simulink model "B"  (R2024a)
settings: Solver=VariableStepAuto  StartTime=0.0  StopTime=10*10^-6  RelTol=1e-3
undefined symbols (not defined in the file): c1, c3, rxDpIndex
libraries: commblkcod2 x64, commofdm x64, commdigbbndam3 x64, commsink2 x1, commseqgen3 x1
(part 1 of 3)
settings Model: Creator=Honest  LastModifiedBy=NEYMAR
settings RTWCC: GPUComputeCapability=3.5

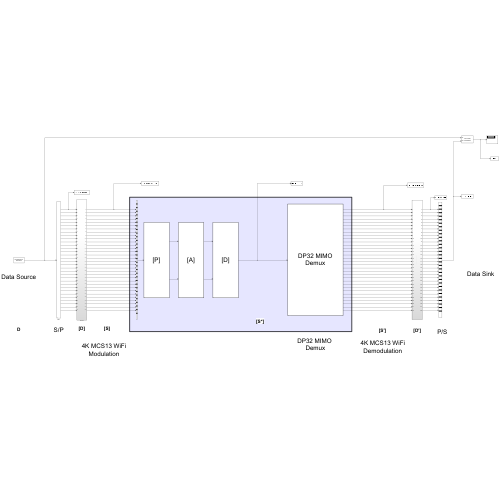
[thumbnail: Simulink's stored preview of the top-level diagram]
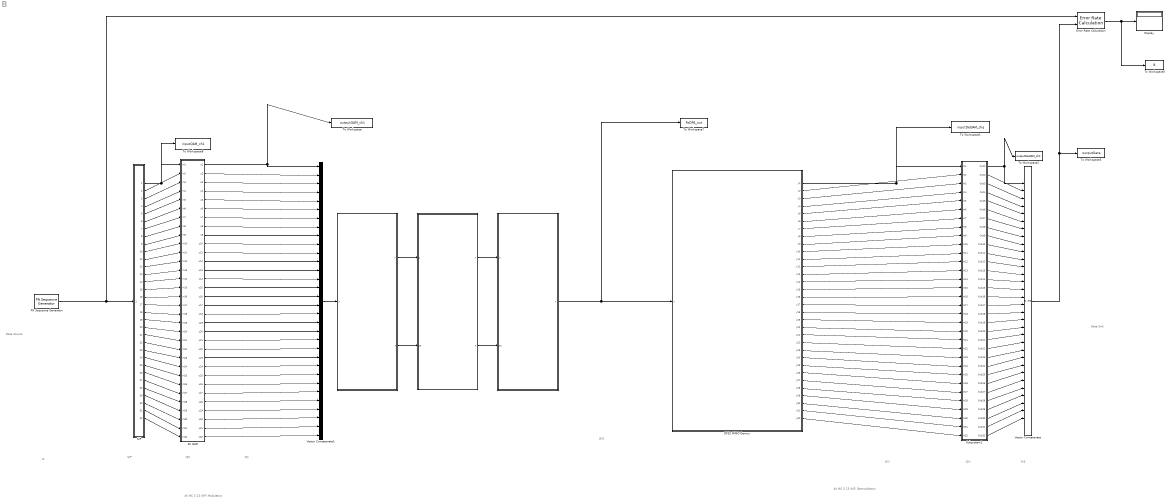
== system B ==
  note: Data Source
  note: D
  note: Data Sink
  note: S/P
  note: 4K MC S 13 WiFi Modulation
  note: P/S
  note: [S']
  note: [D]
  note: [S]
  note: [S*]
  note: [D']
  note: 4K MC S 13 WiFi Demodulation
  " " : MATLAB Function  TreatAsAtomicUnit=on
  " " : MATLAB Function  TreatAsAtomicUnit=on
  " DP32 MIMO Demux" : MATLAB Function  TreatAsAtomicUnit=on
  "    " : MATLAB Function  TreatAsAtomicUnit=on
  4K QAM : Subsystem
  Display : Display
  Error Rate Calculation : commsink2/Error Rate Calculation  N=0  st_delay=0  cp_mode=Entire frame  subframe=[]  PMode=Port  WsName=ErrorVec  RsMode2=off  stop=off  numErr=10000  maxBits=1e8
  PN Sequence Generator : commseqgen3/PN Sequence Generator  poly='z^15 + z^14 + 1'  ini_sta=[0 0 0 0 0 0 0 0 0 0 0 0 0 0 1]  outBitMaskSource=Dialog parameter  shift=0  outVarSiz=off  maxOutSizeMode=Dialog parameter  maxOutSize=[10 1]  Ts=1.0845987*10^-11  sampPerFrame=1254400  reset=off  bitPackedOutputs=off  outDataType=double  numPackedBits=8  bitPackDataSigned=off  bitPackedOutDType=double
  S/P : Subsystem
      mask Display: text(5, 10, 'Serial to Parallel Converter');
  Subsystem1 : Subsystem
  To Workspace : ToWorkspace  VariableName=outputQAM_ch1  SampleTime=-1
      settings: Save2DSignal=2-D array (concatenate along first dimension)
  To Workspace1 : ToWorkspace  VariableName=inputDeQAM_chq  SampleTime=-1
      settings: Save2DSignal=2-D array (concatenate along first dimension)
  To Workspace2 : ToWorkspace  VariableName=outputDeQAM_ch1  SampleTime=-1
      settings: Save2DSignal=2-D array (concatenate along first dimension)
  To Workspace3 : ToWorkspace  VariableName=outputData  SampleTime=-1
      settings: Save2DSignal=2-D array (concatenate along first dimension)
  To Workspace5 : ToWorkspace  VariableName=B  SampleTime=-1
      settings: MaxDataPoints=1  Save2DSignal=2-D array (concatenate along first dimension)
  To Workspace7 : ToWorkspace  VariableName=RxDPA_out  SampleTime=-1
      settings: Save2DSignal=2-D array (concatenate along first dimension)
  To Workspace8 : ToWorkspace  VariableName=inputQAM_ch1  SampleTime=-1
      settings: Save2DSignal=2-D array (concatenate along first dimension)
  Vector Concatenate : Concatenate  NumInputs=32
  Vector Concatenate1 : Concatenate  NumInputs=32
  wires:
  S/P/9(Out9) -> 4K QAM/9(In9)
  4K QAM/23(u23) -> Vector Concatenate1/23
  S/P/17(Out17) -> 4K QAM/17(In17)
  Subsystem1/18(Out18) -> Vector Concatenate/18
  S/P/18(Out18) -> 4K QAM/18(In18)
  Vector Concatenate1/1 -> " "/1(u)
  Subsystem1/12(Out12) -> Vector Concatenate/12
  4K QAM/20(u20) -> Vector Concatenate1/20
  S/P/32(Out32) -> 4K QAM/32(In32)
  Subsystem1/7(Out7) -> Vector Concatenate/7
  Subsystem1/1(Out1) -> Vector Concatenate/1, To Workspace2/1
  Subsystem1/30(Out30) -> Vector Concatenate/30
  4K QAM/26(u26) -> Vector Concatenate1/26
  4K QAM/18(u18) -> Vector Concatenate1/18
  Subsystem1/23(Out23) -> Vector Concatenate/23
  S/P/12(Out12) -> 4K QAM/12(In12)
  4K QAM/19(u19) -> Vector Concatenate1/19
  Subsystem1/26(Out26) -> Vector Concatenate/26
  4K QAM/32(u32) -> Vector Concatenate1/32
  4K QAM/30(u30) -> Vector Concatenate1/30
  4K QAM/28(u28) -> Vector Concatenate1/28
  S/P/13(Out13) -> 4K QAM/13(In13)
  Subsystem1/25(Out25) -> Vector Concatenate/25
  Subsystem1/10(Out10) -> Vector Concatenate/10
  Subsystem1/24(Out24) -> Vector Concatenate/24
  S/P/8(Out8) -> 4K QAM/8(In8)
  Subsystem1/29(Out29) -> Vector Concatenate/29
  Subsystem1/21(Out21) -> Vector Concatenate/21
  Subsystem1/27(Out27) -> Vector Concatenate/27
  Subsystem1/22(Out22) -> Vector Concatenate/22
  4K QAM/31(u31) -> Vector Concatenate1/31
  Subsystem1/28(Out28) -> Vector Concatenate/28
  Subsystem1/32(Out32) -> Vector Concatenate/32
  Subsystem1/6(Out6) -> Vector Concatenate/6
  Subsystem1/20(Out20) -> Vector Concatenate/20
  Subsystem1/8(Out8) -> Vector Concatenate/8
  S/P/21(Out21) -> 4K QAM/21(In21)
  Subsystem1/19(Out19) -> Vector Concatenate/19
  S/P/2(Out2) -> 4K QAM/2(In2)
  Subsystem1/3(Out3) -> Vector Concatenate/3
  Subsystem1/11(Out11) -> Vector Concatenate/11
  Subsystem1/4(Out4) -> Vector Concatenate/4
  S/P/20(Out20) -> 4K QAM/20(In20)
  Subsystem1/13(Out13) -> Vector Concatenate/13
  S/P/29(Out29) -> 4K QAM/29(In29)
  4K QAM/29(u29) -> Vector Concatenate1/29
  S/P/14(Out14) -> 4K QAM/14(In14)
  Subsystem1/14(Out14) -> Vector Concatenate/14
  Subsystem1/9(Out9) -> Vector Concatenate/9
  S/P/23(Out23) -> 4K QAM/23(In23)
  S/P/19(Out19) -> 4K QAM/19(In19)
  Subsystem1/31(Out31) -> Vector Concatenate/31
  S/P/26(Out26) -> 4K QAM/26(In26)
  4K QAM/17(u17) -> Vector Concatenate1/17
  S/P/25(Out25) -> 4K QAM/25(In25)
  S/P/6(Out6) -> 4K QAM/6(In6)
  S/P/22(Out22) -> 4K QAM/22(In22)
  Subsystem1/16(Out16) -> Vector Concatenate/16
  S/P/28(Out28) -> 4K QAM/28(In28)
  S/P/31(Out31) -> 4K QAM/31(In31)
  S/P/27(Out27) -> 4K QAM/27(In27)
  S/P/16(Out16) -> 4K QAM/16(In16)
  Subsystem1/5(Out5) -> Vector Concatenate/5
  S/P/15(Out15) -> 4K QAM/15(In15)
  S/P/10(Out10) -> 4K QAM/10(In10)
  Subsystem1/15(Out15) -> Vector Concatenate/15
  S/P/24(Out24) -> 4K QAM/24(In24)
  S/P/30(Out30) -> 4K QAM/30(In30)
  S/P/3(Out3) -> 4K QAM/3(In3)
  S/P/7(Out7) -> 4K QAM/7(In7)
  S/P/1(Out1) -> 4K QAM/1(In1), To Workspace8/1
  4K QAM/21(u21) -> Vector Concatenate1/21
  S/P/4(Out4) -> 4K QAM/4(In4)
  S/P/5(Out5) -> 4K QAM/5(In5)
  Subsystem1/17(Out17) -> Vector Concatenate/17
  S/P/11(Out11) -> 4K QAM/11(In11)
  Subsystem1/2(Out2) -> Vector Concatenate/2
  Vector Concatenate/1 -> Error Rate Calculation/2, To Workspace3/1
  Error Rate Calculation/1 -> Display/1, To Workspace5/1
  PN Sequence Generator/1 -> Error Rate Calculation/1, S/P/1(In1)
  " DP32 MIMO Demux"/2(y2) -> Subsystem1/2(In2)
  " DP32 MIMO Demux"/3(y3) -> Subsystem1/3(In3)
  " DP32 MIMO Demux"/4(y4) -> Subsystem1/4(In4)
  " DP32 MIMO Demux"/5(y5) -> Subsystem1/5(In5)
  " DP32 MIMO Demux"/6(y6) -> Subsystem1/6(In6)
  " DP32 MIMO Demux"/7(y7) -> Subsystem1/7(In7)
  " DP32 MIMO Demux"/8(y8) -> Subsystem1/8(In8)
  " DP32 MIMO Demux"/9(y9) -> Subsystem1/9(In9)
  " DP32 MIMO Demux"/10(y10) -> Subsystem1/10(In10)
  " DP32 MIMO Demux"/11(y11) -> Subsystem1/11(In11)
  " DP32 MIMO Demux"/12(y12) -> Subsystem1/12(In12)
  " DP32 MIMO Demux"/13(y13) -> Subsystem1/13(In13)
  " DP32 MIMO Demux"/14(y14) -> Subsystem1/14(In14)
  " DP32 MIMO Demux"/15(y15) -> Subsystem1/15(In15)
  " DP32 MIMO Demux"/16(y16) -> Subsystem1/16(In16)
  " DP32 MIMO Demux"/17(y17) -> Subsystem1/17(In17)
  " DP32 MIMO Demux"/18(y18) -> Subsystem1/18(In18)
  " DP32 MIMO Demux"/19(y19) -> Subsystem1/19(In19)
  " DP32 MIMO Demux"/20(y20) -> Subsystem1/20(In20)
  " DP32 MIMO Demux"/21(y21) -> Subsystem1/21(In21)
  " DP32 MIMO Demux"/22(y22) -> Subsystem1/22(In22)
  " DP32 MIMO Demux"/23(y23) -> Subsystem1/23(In23)
  " DP32 MIMO Demux"/24(y24) -> Subsystem1/24(In24)
  " DP32 MIMO Demux"/25(y25) -> Subsystem1/25(In25)
  " DP32 MIMO Demux"/26(y26) -> Subsystem1/26(In26)
  " DP32 MIMO Demux"/27(y27) -> Subsystem1/27(In27)
  " DP32 MIMO Demux"/28(y28) -> Subsystem1/28(In28)
  " DP32 MIMO Demux"/29(y29) -> Subsystem1/29(In29)
  " DP32 MIMO Demux"/30(y30) -> Subsystem1/30(In30)
  " DP32 MIMO Demux"/31(y31) -> Subsystem1/31(In31)
  " DP32 MIMO Demux"/32(y32) -> Subsystem1/32(In32)
  4K QAM/2(u2) -> Vector Concatenate1/2
  4K QAM/5(u5) -> Vector Concatenate1/5
  4K QAM/6(u6) -> Vector Concatenate1/6
  4K QAM/7(u7) -> Vector Concatenate1/7
  4K QAM/8(u8) -> Vector Concatenate1/8
  4K QAM/9(u9) -> Vector Concatenate1/9
  4K QAM/10(u10) -> Vector Concatenate1/10
  4K QAM/11(u11) -> Vector Concatenate1/11
  4K QAM/12(u12) -> Vector Concatenate1/12
  4K QAM/13(u13) -> Vector Concatenate1/13
  4K QAM/14(u14) -> Vector Concatenate1/14
  4K QAM/15(u15) -> Vector Concatenate1/15
  4K QAM/16(u16) -> Vector Concatenate1/16
  4K QAM/24(u24) -> Vector Concatenate1/24
  4K QAM/3(u3) -> Vector Concatenate1/3
  4K QAM/4(u4) -> Vector Concatenate1/4
  4K QAM/22(u22) -> Vector Concatenate1/22
  4K QAM/25(u25) -> Vector Concatenate1/25
  4K QAM/27(u27) -> Vector Concatenate1/27
  " DP32 MIMO Demux"/1(y1) -> Subsystem1/1(In1), To Workspace1/1
  4K QAM/1(u1) -> To Workspace/1, Vector Concatenate1/1
  " "/1(y) -> "    "/1(u)
  "    "/1(y) -> " "/1(u)
  " "/1(y) -> To Workspace7/1, " DP32 MIMO Demux"/1(u)
  " "/2(s) -> "    "/2(ss)
  "    "/2(s) -> " "/2(ss)

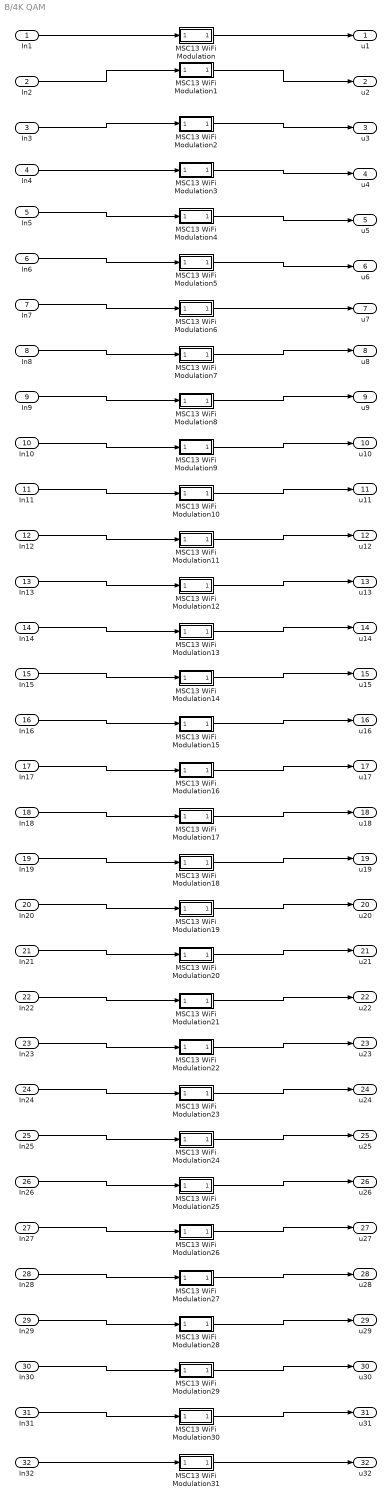
== system B/4K QAM ==
  In1 : Inport
  In2 : Inport  Port=2
  In3 : Inport  Port=3
  In4 : Inport  Port=4
  In5 : Inport  Port=5
  In6 : Inport  Port=6
  In7 : Inport  Port=7
  In8 : Inport  Port=8
  In9 : Inport  Port=9
  In10 : Inport  Port=10
  In11 : Inport  Port=11
  In12 : Inport  Port=12
  In13 : Inport  Port=13
  In14 : Inport  Port=14
  In15 : Inport  Port=15
  In16 : Inport  Port=16
  In17 : Inport  Port=17
  In18 : Inport  Port=18
  In19 : Inport  Port=19
  In20 : Inport  Port=20
  In21 : Inport  Port=21
  In22 : Inport  Port=22
  In23 : Inport  Port=23
  In24 : Inport  Port=24
  In25 : Inport  Port=25
  In26 : Inport  Port=26
  In27 : Inport  Port=27
  In28 : Inport  Port=28
  In29 : Inport  Port=29
  In30 : Inport  Port=30
  In31 : Inport  Port=31
  In32 : Inport  Port=32
  MSC13 WiFi Modulation : Subsystem
  MSC13 WiFi Modulation1 : Subsystem
  MSC13 WiFi Modulation10 : Subsystem
  MSC13 WiFi Modulation11 : Subsystem
  MSC13 WiFi Modulation12 : Subsystem
  MSC13 WiFi Modulation13 : Subsystem
  MSC13 WiFi Modulation14 : Subsystem
  MSC13 WiFi Modulation15 : Subsystem
  MSC13 WiFi Modulation16 : Subsystem
  MSC13 WiFi Modulation17 : Subsystem
  MSC13 WiFi Modulation18 : Subsystem
  MSC13 WiFi Modulation19 : Subsystem
  MSC13 WiFi Modulation2 : Subsystem
  MSC13 WiFi Modulation20 : Subsystem
  MSC13 WiFi Modulation21 : Subsystem
  MSC13 WiFi Modulation22 : Subsystem
  MSC13 WiFi Modulation23 : Subsystem
  MSC13 WiFi Modulation24 : Subsystem
  MSC13 WiFi Modulation25 : Subsystem
  MSC13 WiFi Modulation26 : Subsystem
  MSC13 WiFi Modulation27 : Subsystem
  MSC13 WiFi Modulation28 : Subsystem
  MSC13 WiFi Modulation29 : Subsystem
  MSC13 WiFi Modulation3 : Subsystem
  MSC13 WiFi Modulation30 : Subsystem
  MSC13 WiFi Modulation31 : Subsystem
  MSC13 WiFi Modulation4 : Subsystem
  MSC13 WiFi Modulation5 : Subsystem
  MSC13 WiFi Modulation6 : Subsystem
  MSC13 WiFi Modulation7 : Subsystem
  MSC13 WiFi Modulation8 : Subsystem
  MSC13 WiFi Modulation9 : Subsystem
  u1 : Outport
  u2 : Outport  Port=2
  u3 : Outport  Port=3
  u4 : Outport  Port=4
  u5 : Outport  Port=5
  u6 : Outport  Port=6
  u7 : Outport  Port=7
  u8 : Outport  Port=8
  u9 : Outport  Port=9
  u10 : Outport  Port=10
  u11 : Outport  Port=11
  u12 : Outport  Port=12
  u13 : Outport  Port=13
  u14 : Outport  Port=14
  u15 : Outport  Port=15
  u16 : Outport  Port=16
  u17 : Outport  Port=17
  u18 : Outport  Port=18
  u19 : Outport  Port=19
  u20 : Outport  Port=20
  u21 : Outport  Port=21
  u22 : Outport  Port=22
  u23 : Outport  Port=23
  u24 : Outport  Port=24
  u25 : Outport  Port=25
  u26 : Outport  Port=26
  u27 : Outport  Port=27
  u28 : Outport  Port=28
  u29 : Outport  Port=29
  u30 : Outport  Port=30
  u31 : Outport  Port=31
  u32 : Outport  Port=32
  wires:
  In1/1 -> MSC13 WiFi Modulation/1(In1)
  MSC13 WiFi Modulation/1(Out1) -> u1/1
  In2/1 -> MSC13 WiFi Modulation1/1(In1)
  MSC13 WiFi Modulation1/1(Out1) -> u2/1
  In32/1 -> MSC13 WiFi Modulation31/1(In1)
  In31/1 -> MSC13 WiFi Modulation30/1(In1)
  In30/1 -> MSC13 WiFi Modulation29/1(In1)
  In27/1 -> MSC13 WiFi Modulation26/1(In1)
  In28/1 -> MSC13 WiFi Modulation27/1(In1)
  In29/1 -> MSC13 WiFi Modulation28/1(In1)
  In26/1 -> MSC13 WiFi Modulation25/1(In1)
  In25/1 -> MSC13 WiFi Modulation24/1(In1)
  In24/1 -> MSC13 WiFi Modulation23/1(In1)
  In23/1 -> MSC13 WiFi Modulation22/1(In1)
  In22/1 -> MSC13 WiFi Modulation21/1(In1)
  In21/1 -> MSC13 WiFi Modulation20/1(In1)
  In20/1 -> MSC13 WiFi Modulation19/1(In1)
  In19/1 -> MSC13 WiFi Modulation18/1(In1)
  In18/1 -> MSC13 WiFi Modulation17/1(In1)
  In17/1 -> MSC13 WiFi Modulation16/1(In1)
  In16/1 -> MSC13 WiFi Modulation15/1(In1)
  In15/1 -> MSC13 WiFi Modulation14/1(In1)
  In14/1 -> MSC13 WiFi Modulation13/1(In1)
  In13/1 -> MSC13 WiFi Modulation12/1(In1)
  In12/1 -> MSC13 WiFi Modulation11/1(In1)
  In11/1 -> MSC13 WiFi Modulation10/1(In1)
  In10/1 -> MSC13 WiFi Modulation9/1(In1)
  In9/1 -> MSC13 WiFi Modulation8/1(In1)
  In8/1 -> MSC13 WiFi Modulation7/1(In1)
  In7/1 -> MSC13 WiFi Modulation6/1(In1)
  In6/1 -> MSC13 WiFi Modulation5/1(In1)
  In4/1 -> MSC13 WiFi Modulation3/1(In1)
  In3/1 -> MSC13 WiFi Modulation2/1(In1)
  In5/1 -> MSC13 WiFi Modulation4/1(In1)
  MSC13 WiFi Modulation2/1(Out1) -> u3/1
  MSC13 WiFi Modulation3/1(Out1) -> u4/1
  MSC13 WiFi Modulation5/1(Out1) -> u6/1
  MSC13 WiFi Modulation4/1(Out1) -> u5/1
  MSC13 WiFi Modulation6/1(Out1) -> u7/1
  MSC13 WiFi Modulation7/1(Out1) -> u8/1
  MSC13 WiFi Modulation8/1(Out1) -> u9/1
  MSC13 WiFi Modulation9/1(Out1) -> u10/1
  MSC13 WiFi Modulation10/1(Out1) -> u11/1
  MSC13 WiFi Modulation11/1(Out1) -> u12/1
  MSC13 WiFi Modulation12/1(Out1) -> u13/1
  MSC13 WiFi Modulation13/1(Out1) -> u14/1
  MSC13 WiFi Modulation14/1(Out1) -> u15/1
  MSC13 WiFi Modulation15/1(Out1) -> u16/1
  MSC13 WiFi Modulation16/1(Out1) -> u17/1
  MSC13 WiFi Modulation17/1(Out1) -> u18/1
  MSC13 WiFi Modulation18/1(Out1) -> u19/1
  MSC13 WiFi Modulation19/1(Out1) -> u20/1
  MSC13 WiFi Modulation20/1(Out1) -> u21/1
  MSC13 WiFi Modulation21/1(Out1) -> u22/1
  MSC13 WiFi Modulation22/1(Out1) -> u23/1
  MSC13 WiFi Modulation23/1(Out1) -> u24/1
  MSC13 WiFi Modulation24/1(Out1) -> u25/1
  MSC13 WiFi Modulation25/1(Out1) -> u26/1
  MSC13 WiFi Modulation26/1(Out1) -> u27/1
  MSC13 WiFi Modulation27/1(Out1) -> u28/1
  MSC13 WiFi Modulation28/1(Out1) -> u29/1
  MSC13 WiFi Modulation29/1(Out1) -> u30/1
  MSC13 WiFi Modulation30/1(Out1) -> u31/1
  MSC13 WiFi Modulation31/1(Out1) -> u32/1

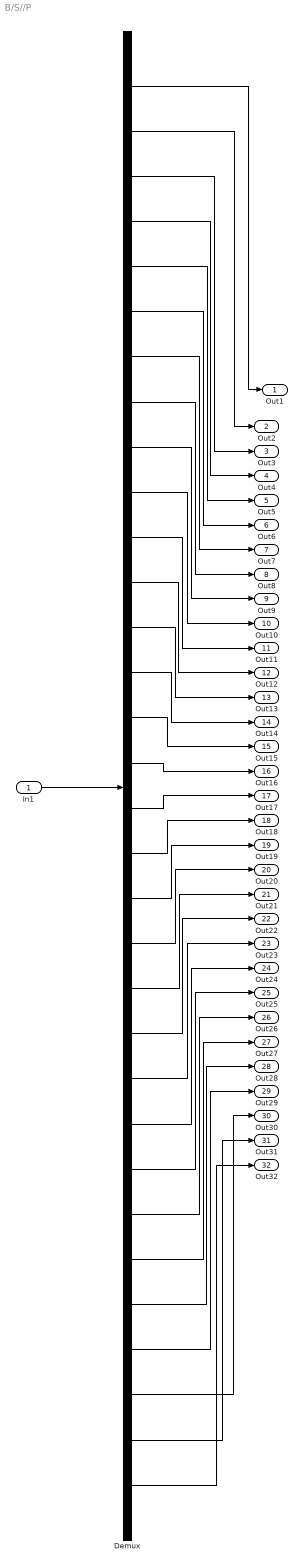
== system B/S//P ==
  In1 : Inport
  Demux : Demux  Outputs=32
  Out1 : Outport
  Out2 : Outport  Port=2
  Out3 : Outport  Port=3
  Out4 : Outport  Port=4
  Out5 : Outport  Port=5
  Out6 : Outport  Port=6
  Out7 : Outport  Port=7
  Out8 : Outport  Port=8
  Out9 : Outport  Port=9
  Out10 : Outport  Port=10
  Out11 : Outport  Port=11
  Out12 : Outport  Port=12
  Out13 : Outport  Port=13
  Out14 : Outport  Port=14
  Out15 : Outport  Port=15
  Out16 : Outport  Port=16
  Out17 : Outport  Port=17
  Out18 : Outport  Port=18
  Out19 : Outport  Port=19
  Out20 : Outport  Port=20
  Out21 : Outport  Port=21
  Out22 : Outport  Port=22
  Out23 : Outport  Port=23
  Out24 : Outport  Port=24
  Out25 : Outport  Port=25
  Out26 : Outport  Port=26
  Out27 : Outport  Port=27
  Out28 : Outport  Port=28
  Out29 : Outport  Port=29
  Out30 : Outport  Port=30
  Out31 : Outport  Port=31
  Out32 : Outport  Port=32
  wires:
  Demux/28 -> Out28/1
  Demux/2 -> Out2/1
  Demux/16 -> Out16/1
  In1/1 -> Demux/1
  Demux/13 -> Out13/1
  Demux/6 -> Out6/1
  Demux/7 -> Out7/1
  Demux/21 -> Out21/1
  Demux/3 -> Out3/1
  Demux/11 -> Out11/1
  Demux/1 -> Out1/1
  Demux/20 -> Out20/1
  Demux/5 -> Out5/1
  Demux/4 -> Out4/1
  Demux/8 -> Out8/1
  Demux/9 -> Out9/1
  Demux/12 -> Out12/1
  Demux/14 -> Out14/1
  Demux/29 -> Out29/1
  Demux/15 -> Out15/1
  Demux/17 -> Out17/1
  Demux/18 -> Out18/1
  Demux/10 -> Out10/1
  Demux/22 -> Out22/1
  Demux/19 -> Out19/1
  Demux/23 -> Out23/1
  Demux/30 -> Out30/1
  Demux/27 -> Out27/1
  Demux/25 -> Out25/1
  Demux/26 -> Out26/1
  Demux/24 -> Out24/1
  Demux/31 -> Out31/1
  Demux/32 -> Out32/1

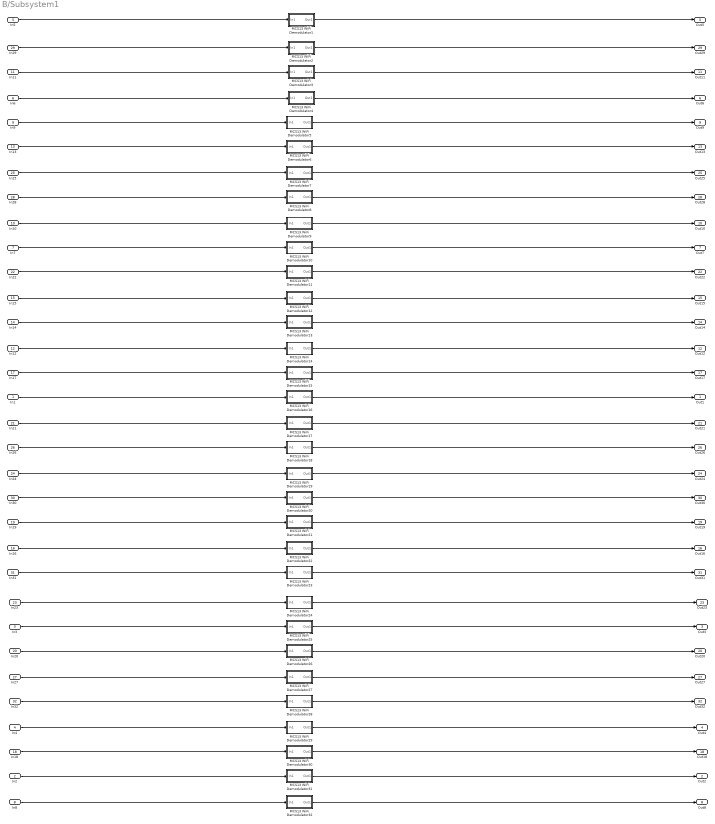
== system B/Subsystem1 ==
  In1 : Inport
  In2 : Inport  Port=2
  In3 : Inport  Port=3
  In4 : Inport  Port=4
  In5 : Inport  Port=5
  In6 : Inport  Port=6
  In7 : Inport  Port=7
  In8 : Inport  Port=8
  In9 : Inport  Port=9
  In10 : Inport  Port=10
  In11 : Inport  Port=11
  In12 : Inport  Port=12
  In13 : Inport  Port=13
  In14 : Inport  Port=14
  In15 : Inport  Port=15
  In16 : Inport  Port=16
  In17 : Inport  Port=17
  In18 : Inport  Port=18
  In19 : Inport  Port=19
  In20 : Inport  Port=20
  In21 : Inport  Port=21
  In22 : Inport  Port=22
  In23 : Inport  Port=23
  In24 : Inport  Port=24
  In25 : Inport  Port=25
  In26 : Inport  Port=26
  In27 : Inport  Port=27
  In28 : Inport  Port=28
  In29 : Inport  Port=29
  In30 : Inport  Port=30
  In31 : Inport  Port=31
  In32 : Inport  Port=32
  MCS13 WiFi Demodulator1 : Subsystem
  MCS13 WiFi Demodulator10 : Subsystem
  MCS13 WiFi Demodulator11 : Subsystem
  MCS13 WiFi Demodulator12 : Subsystem
  MCS13 WiFi Demodulator13 : Subsystem
  MCS13 WiFi Demodulator14 : Subsystem
  MCS13 WiFi Demodulator15 : Subsystem
  MCS13 WiFi Demodulator16 : Subsystem
  MCS13 WiFi Demodulator17 : Subsystem
  MCS13 WiFi Demodulator18 : Subsystem
  MCS13 WiFi Demodulator19 : Subsystem
  MCS13 WiFi Demodulator2 : Subsystem
  MCS13 WiFi Demodulator20 : Subsystem
  MCS13 WiFi Demodulator21 : Subsystem
  MCS13 WiFi Demodulator22 : Subsystem
  MCS13 WiFi Demodulator23 : Subsystem
  MCS13 WiFi Demodulator24 : Subsystem
  MCS13 WiFi Demodulator25 : Subsystem
  MCS13 WiFi Demodulator26 : Subsystem
  MCS13 WiFi Demodulator27 : Subsystem
  MCS13 WiFi Demodulator28 : Subsystem
  MCS13 WiFi Demodulator29 : Subsystem
  MCS13 WiFi Demodulator3 : Subsystem
  MCS13 WiFi Demodulator30 : Subsystem
  MCS13 WiFi Demodulator31 : Subsystem
  MCS13 WiFi Demodulator32 : Subsystem
  MCS13 WiFi Demodulator4 : Subsystem
  MCS13 WiFi Demodulator5 : Subsystem
  MCS13 WiFi Demodulator6 : Subsystem
  MCS13 WiFi Demodulator7 : Subsystem
  MCS13 WiFi Demodulator8 : Subsystem
  MCS13 WiFi Demodulator9 : Subsystem
  Out1 : Outport
  Out2 : Outport  Port=2
  Out3 : Outport  Port=3
  Out4 : Outport  Port=4
  Out5 : Outport  Port=5
  Out6 : Outport  Port=6
  Out7 : Outport  Port=7
  Out8 : Outport  Port=8
  Out9 : Outport  Port=9
  Out10 : Outport  Port=10
  Out11 : Outport  Port=11
  Out12 : Outport  Port=12
  Out13 : Outport  Port=13
  Out14 : Outport  Port=14
  Out15 : Outport  Port=15
  Out16 : Outport  Port=16
  Out17 : Outport  Port=17
  Out18 : Outport  Port=18
  Out19 : Outport  Port=19
  Out20 : Outport  Port=20
  Out21 : Outport  Port=21
  Out22 : Outport  Port=22
  Out23 : Outport  Port=23
  Out24 : Outport  Port=24
  Out25 : Outport  Port=25
  Out26 : Outport  Port=26
  Out27 : Outport  Port=27
  Out28 : Outport  Port=28
  Out29 : Outport  Port=29
  Out30 : Outport  Port=30
  Out31 : Outport  Port=31
  Out32 : Outport  Port=32
  wires:
  MCS13 WiFi Demodulator16/1(Out1) -> Out1/1
  MCS13 WiFi Demodulator31/1(Out1) -> Out2/1
  MCS13 WiFi Demodulator25/1(Out1) -> Out3/1
  MCS13 WiFi Demodulator29/1(Out1) -> Out4/1
  MCS13 WiFi Demodulator1/1(Out1) -> Out5/1
  MCS13 WiFi Demodulator4/1(Out1) -> Out6/1
  MCS13 WiFi Demodulator10/1(Out1) -> Out7/1
  MCS13 WiFi Demodulator32/1(Out1) -> Out8/1
  MCS13 WiFi Demodulator5/1(Out1) -> Out9/1
  MCS13 WiFi Demodulator9/1(Out1) -> Out10/1
  MCS13 WiFi Demodulator3/1(Out1) -> Out11/1
  MCS13 WiFi Demodulator14/1(Out1) -> Out12/1
  MCS13 WiFi Demodulator6/1(Out1) -> Out13/1
  MCS13 WiFi Demodulator13/1(Out1) -> Out14/1
  MCS13 WiFi Demodulator12/1(Out1) -> Out15/1
  MCS13 WiFi Demodulator22/1(Out1) -> Out16/1
  MCS13 WiFi Demodulator15/1(Out1) -> Out17/1
  MCS13 WiFi Demodulator30/1(Out1) -> Out18/1
  MCS13 WiFi Demodulator21/1(Out1) -> Out19/1
  MCS13 WiFi Demodulator26/1(Out1) -> Out20/1
  MCS13 WiFi Demodulator17/1(Out1) -> Out21/1
  MCS13 WiFi Demodulator11/1(Out1) -> Out22/1
  MCS13 WiFi Demodulator24/1(Out1) -> Out23/1
  MCS13 WiFi Demodulator19/1(Out1) -> Out24/1
  MCS13 WiFi Demodulator7/1(Out1) -> Out25/1
  MCS13 WiFi Demodulator18/1(Out1) -> Out26/1
  MCS13 WiFi Demodulator27/1(Out1) -> Out27/1
  MCS13 WiFi Demodulator8/1(Out1) -> Out28/1
  MCS13 WiFi Demodulator2/1(Out1) -> Out29/1
  MCS13 WiFi Demodulator20/1(Out1) -> Out30/1
  MCS13 WiFi Demodulator23/1(Out1) -> Out31/1
  MCS13 WiFi Demodulator28/1(Out1) -> Out32/1
  In19/1 -> MCS13 WiFi Demodulator21/1(In1)
  In3/1 -> MCS13 WiFi Demodulator25/1(In1)
  In31/1 -> MCS13 WiFi Demodulator23/1(In1)
  In2/1 -> MCS13 WiFi Demodulator31/1(In1)
  In13/1 -> MCS13 WiFi Demodulator6/1(In1)
  In1/1 -> MCS13 WiFi Demodulator16/1(In1)
  In18/1 -> MCS13 WiFi Demodulator30/1(In1)
  In10/1 -> MCS13 WiFi Demodulator9/1(In1)
  In4/1 -> MCS13 WiFi Demodulator29/1(In1)
  In5/1 -> MCS13 WiFi Demodulator1/1(In1)
  In28/1 -> MCS13 WiFi Demodulator8/1(In1)
  In21/1 -> MCS13 WiFi Demodulator17/1(In1)
  In14/1 -> MCS13 WiFi Demodulator13/1(In1)
  In15/1 -> MCS13 WiFi Demodulator12/1(In1)
  In20/1 -> MCS13 WiFi Demodulator26/1(In1)
  In11/1 -> MCS13 WiFi Demodulator3/1(In1)
  In22/1 -> MCS13 WiFi Demodulator11/1(In1)
  In7/1 -> MCS13 WiFi Demodulator10/1(In1)
  In23/1 -> MCS13 WiFi Demodulator24/1(In1)
  In12/1 -> MCS13 WiFi Demodulator14/1(In1)
  In30/1 -> MCS13 WiFi Demodulator20/1(In1)
  In9/1 -> MCS13 WiFi Demodulator5/1(In1)
  In32/1 -> MCS13 WiFi Demodulator28/1(In1)
  In29/1 -> MCS13 WiFi Demodulator2/1(In1)
  In16/1 -> MCS13 WiFi Demodulator22/1(In1)
  In26/1 -> MCS13 WiFi Demodulator18/1(In1)
  In24/1 -> MCS13 WiFi Demodulator19/1(In1)
  In25/1 -> MCS13 WiFi Demodulator7/1(In1)
  In8/1 -> MCS13 WiFi Demodulator32/1(In1)
  In6/1 -> MCS13 WiFi Demodulator4/1(In1)
  In27/1 -> MCS13 WiFi Demodulator27/1(In1)
  In17/1 -> MCS13 WiFi Demodulator15/1(In1)

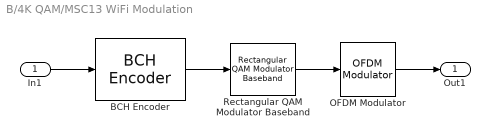
== system B/4K QAM/MSC13 WiFi Modulation ==
  In1 : Inport
  BCH Encoder : commblkcod2/BCH Encoder  n=47040  k=39200  specShortening=off  shortenedK=5  specGenPoly=off  genPoly='X^10 + X^8 + X^5 + X^4 + X^2 + X + 1'  specPrimPoly=off  prPoly='X^4 + X + 1'  specDisableGenCheck=off  specPuncture=off  punctVec=[ones(8,1); zeros(2,1)]
  OFDM Modulator : commofdm/OFDM Modulator  StatePerturbationForJacobian=1.0e-05  FFTLength=4096  NumGuardBandCarriers=[88; 88]  InsertDCNull=off  PilotInputPort=off  PilotCarrierIndices=[52;104;156;208;260]  CyclicPrefixLength=0  Windowing=off  WindowLength=1  OversamplingFactor=1  NumSymbols=1  NumTransmitAntennas=1  SimulateUsing=Interpreted execution
  Rectangular QAM Modulator Baseband : commdigbbndam3/Rectangular QAM Modulator Baseband  M=4096  InType=Bit  Enc=Gray  Mapping=[0:15]  PowType=Min. distance between symbols  MinDist=2  AvgPow=1  PeakPow=1  Ph=0  outDtype=double  outWordLen=16  outUDDataType=sfix(16)  outFracLenMode=Best precision  outFracLen=15  outDataTypeStr=double  outLastDataTypeStr=double
  Out1 : Outport
  wires:
  Rectangular QAM Modulator Baseband/1 -> OFDM Modulator/1
  OFDM Modulator/1 -> Out1/1
  BCH Encoder/1 -> Rectangular QAM Modulator Baseband/1
  In1/1 -> BCH Encoder/1

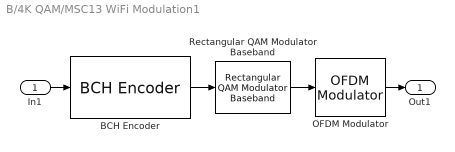
== system B/4K QAM/MSC13 WiFi Modulation1 ==
  In1 : Inport
  BCH Encoder : commblkcod2/BCH Encoder  n=47040  k=39200  specShortening=off  shortenedK=5  specGenPoly=off  genPoly='X^10 + X^8 + X^5 + X^4 + X^2 + X + 1'  specPrimPoly=off  prPoly='X^4 + X + 1'  specDisableGenCheck=off  specPuncture=off  punctVec=[ones(8,1); zeros(2,1)]
  OFDM Modulator : commofdm/OFDM Modulator  StatePerturbationForJacobian=1.0e-05  FFTLength=4096  NumGuardBandCarriers=[88; 88]  InsertDCNull=off  PilotInputPort=off  PilotCarrierIndices=[52;104;156;208;260]  CyclicPrefixLength=0  Windowing=off  WindowLength=1  OversamplingFactor=1  NumSymbols=1  NumTransmitAntennas=1  SimulateUsing=Interpreted execution
  Rectangular QAM Modulator Baseband : commdigbbndam3/Rectangular QAM Modulator Baseband  M=4096  InType=Bit  Enc=Gray  Mapping=[0:15]  PowType=Min. distance between symbols  MinDist=2  AvgPow=1  PeakPow=1  Ph=0  outDtype=double  outWordLen=16  outUDDataType=sfix(16)  outFracLenMode=Best precision  outFracLen=15  outDataTypeStr=double  outLastDataTypeStr=double
  Out1 : Outport
  wires:
  Rectangular QAM Modulator Baseband/1 -> OFDM Modulator/1
  OFDM Modulator/1 -> Out1/1
  BCH Encoder/1 -> Rectangular QAM Modulator Baseband/1
  In1/1 -> BCH Encoder/1

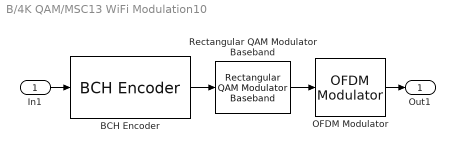
== system B/4K QAM/MSC13 WiFi Modulation10 ==
  In1 : Inport
  BCH Encoder : commblkcod2/BCH Encoder  n=47040  k=39200  specShortening=off  shortenedK=5  specGenPoly=off  genPoly='X^10 + X^8 + X^5 + X^4 + X^2 + X + 1'  specPrimPoly=off  prPoly='X^4 + X + 1'  specDisableGenCheck=off  specPuncture=off  punctVec=[ones(8,1); zeros(2,1)]
  OFDM Modulator : commofdm/OFDM Modulator  StatePerturbationForJacobian=1.0e-05  FFTLength=4096  NumGuardBandCarriers=[88; 88]  InsertDCNull=off  PilotInputPort=off  PilotCarrierIndices=[52;104;156;208;260]  CyclicPrefixLength=0  Windowing=off  WindowLength=1  OversamplingFactor=1  NumSymbols=1  NumTransmitAntennas=1  SimulateUsing=Interpreted execution
  Rectangular QAM Modulator Baseband : commdigbbndam3/Rectangular QAM Modulator Baseband  M=4096  InType=Bit  Enc=Gray  Mapping=[0:15]  PowType=Min. distance between symbols  MinDist=2  AvgPow=1  PeakPow=1  Ph=0  outDtype=double  outWordLen=16  outUDDataType=sfix(16)  outFracLenMode=Best precision  outFracLen=15  outDataTypeStr=double  outLastDataTypeStr=double
  Out1 : Outport
  wires:
  Rectangular QAM Modulator Baseband/1 -> OFDM Modulator/1
  OFDM Modulator/1 -> Out1/1
  BCH Encoder/1 -> Rectangular QAM Modulator Baseband/1
  In1/1 -> BCH Encoder/1

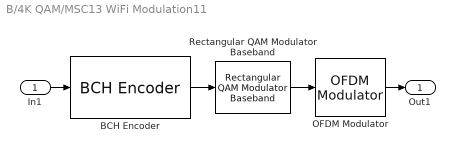
== system B/4K QAM/MSC13 WiFi Modulation11 ==
  In1 : Inport
  BCH Encoder : commblkcod2/BCH Encoder  n=47040  k=39200  specShortening=off  shortenedK=5  specGenPoly=off  genPoly='X^10 + X^8 + X^5 + X^4 + X^2 + X + 1'  specPrimPoly=off  prPoly='X^4 + X + 1'  specDisableGenCheck=off  specPuncture=off  punctVec=[ones(8,1); zeros(2,1)]
  OFDM Modulator : commofdm/OFDM Modulator  StatePerturbationForJacobian=1.0e-05  FFTLength=4096  NumGuardBandCarriers=[88; 88]  InsertDCNull=off  PilotInputPort=off  PilotCarrierIndices=[52;104;156;208;260]  CyclicPrefixLength=0  Windowing=off  WindowLength=1  OversamplingFactor=1  NumSymbols=1  NumTransmitAntennas=1  SimulateUsing=Interpreted execution
  Rectangular QAM Modulator Baseband : commdigbbndam3/Rectangular QAM Modulator Baseband  M=4096  InType=Bit  Enc=Gray  Mapping=[0:15]  PowType=Min. distance between symbols  MinDist=2  AvgPow=1  PeakPow=1  Ph=0  outDtype=double  outWordLen=16  outUDDataType=sfix(16)  outFracLenMode=Best precision  outFracLen=15  outDataTypeStr=double  outLastDataTypeStr=double
  Out1 : Outport
  wires:
  Rectangular QAM Modulator Baseband/1 -> OFDM Modulator/1
  OFDM Modulator/1 -> Out1/1
  BCH Encoder/1 -> Rectangular QAM Modulator Baseband/1
  In1/1 -> BCH Encoder/1

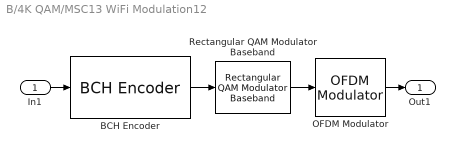
== system B/4K QAM/MSC13 WiFi Modulation12 ==
  In1 : Inport
  BCH Encoder : commblkcod2/BCH Encoder  n=47040  k=39200  specShortening=off  shortenedK=5  specGenPoly=off  genPoly='X^10 + X^8 + X^5 + X^4 + X^2 + X + 1'  specPrimPoly=off  prPoly='X^4 + X + 1'  specDisableGenCheck=off  specPuncture=off  punctVec=[ones(8,1); zeros(2,1)]
  OFDM Modulator : commofdm/OFDM Modulator  StatePerturbationForJacobian=1.0e-05  FFTLength=4096  NumGuardBandCarriers=[88; 88]  InsertDCNull=off  PilotInputPort=off  PilotCarrierIndices=[52;104;156;208;260]  CyclicPrefixLength=0  Windowing=off  WindowLength=1  OversamplingFactor=1  NumSymbols=1  NumTransmitAntennas=1  SimulateUsing=Interpreted execution
  Rectangular QAM Modulator Baseband : commdigbbndam3/Rectangular QAM Modulator Baseband  M=4096  InType=Bit  Enc=Gray  Mapping=[0:15]  PowType=Min. distance between symbols  MinDist=2  AvgPow=1  PeakPow=1  Ph=0  outDtype=double  outWordLen=16  outUDDataType=sfix(16)  outFracLenMode=Best precision  outFracLen=15  outDataTypeStr=double  outLastDataTypeStr=double
  Out1 : Outport
  wires:
  Rectangular QAM Modulator Baseband/1 -> OFDM Modulator/1
  OFDM Modulator/1 -> Out1/1
  BCH Encoder/1 -> Rectangular QAM Modulator Baseband/1
  In1/1 -> BCH Encoder/1

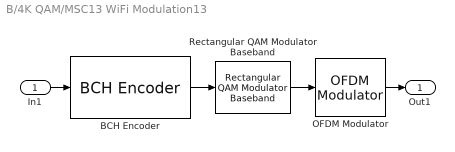
== system B/4K QAM/MSC13 WiFi Modulation13 ==
  In1 : Inport
  BCH Encoder : commblkcod2/BCH Encoder  n=47040  k=39200  specShortening=off  shortenedK=5  specGenPoly=off  genPoly='X^10 + X^8 + X^5 + X^4 + X^2 + X + 1'  specPrimPoly=off  prPoly='X^4 + X + 1'  specDisableGenCheck=off  specPuncture=off  punctVec=[ones(8,1); zeros(2,1)]
  OFDM Modulator : commofdm/OFDM Modulator  StatePerturbationForJacobian=1.0e-05  FFTLength=4096  NumGuardBandCarriers=[88; 88]  InsertDCNull=off  PilotInputPort=off  PilotCarrierIndices=[52;104;156;208;260]  CyclicPrefixLength=0  Windowing=off  WindowLength=1  OversamplingFactor=1  NumSymbols=1  NumTransmitAntennas=1  SimulateUsing=Interpreted execution
  Rectangular QAM Modulator Baseband : commdigbbndam3/Rectangular QAM Modulator Baseband  M=4096  InType=Bit  Enc=Gray  Mapping=[0:15]  PowType=Min. distance between symbols  MinDist=2  AvgPow=1  PeakPow=1  Ph=0  outDtype=double  outWordLen=16  outUDDataType=sfix(16)  outFracLenMode=Best precision  outFracLen=15  outDataTypeStr=double  outLastDataTypeStr=double
  Out1 : Outport
  wires:
  Rectangular QAM Modulator Baseband/1 -> OFDM Modulator/1
  OFDM Modulator/1 -> Out1/1
  BCH Encoder/1 -> Rectangular QAM Modulator Baseband/1
  In1/1 -> BCH Encoder/1

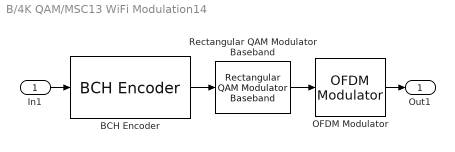
== system B/4K QAM/MSC13 WiFi Modulation14 ==
  In1 : Inport
  BCH Encoder : commblkcod2/BCH Encoder  n=47040  k=39200  specShortening=off  shortenedK=5  specGenPoly=off  genPoly='X^10 + X^8 + X^5 + X^4 + X^2 + X + 1'  specPrimPoly=off  prPoly='X^4 + X + 1'  specDisableGenCheck=off  specPuncture=off  punctVec=[ones(8,1); zeros(2,1)]
  OFDM Modulator : commofdm/OFDM Modulator  StatePerturbationForJacobian=1.0e-05  FFTLength=4096  NumGuardBandCarriers=[88; 88]  InsertDCNull=off  PilotInputPort=off  PilotCarrierIndices=[52;104;156;208;260]  CyclicPrefixLength=0  Windowing=off  WindowLength=1  OversamplingFactor=1  NumSymbols=1  NumTransmitAntennas=1  SimulateUsing=Interpreted execution
  Rectangular QAM Modulator Baseband : commdigbbndam3/Rectangular QAM Modulator Baseband  M=4096  InType=Bit  Enc=Gray  Mapping=[0:15]  PowType=Min. distance between symbols  MinDist=2  AvgPow=1  PeakPow=1  Ph=0  outDtype=double  outWordLen=16  outUDDataType=sfix(16)  outFracLenMode=Best precision  outFracLen=15  outDataTypeStr=double  outLastDataTypeStr=double
  Out1 : Outport
  wires:
  Rectangular QAM Modulator Baseband/1 -> OFDM Modulator/1
  OFDM Modulator/1 -> Out1/1
  BCH Encoder/1 -> Rectangular QAM Modulator Baseband/1
  In1/1 -> BCH Encoder/1

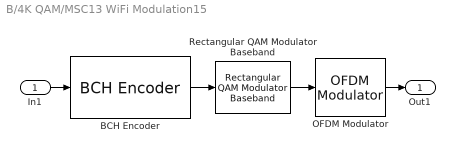
== system B/4K QAM/MSC13 WiFi Modulation15 ==
  In1 : Inport
  BCH Encoder : commblkcod2/BCH Encoder  n=47040  k=39200  specShortening=off  shortenedK=5  specGenPoly=off  genPoly='X^10 + X^8 + X^5 + X^4 + X^2 + X + 1'  specPrimPoly=off  prPoly='X^4 + X + 1'  specDisableGenCheck=off  specPuncture=off  punctVec=[ones(8,1); zeros(2,1)]
  OFDM Modulator : commofdm/OFDM Modulator  StatePerturbationForJacobian=1.0e-05  FFTLength=4096  NumGuardBandCarriers=[88; 88]  InsertDCNull=off  PilotInputPort=off  PilotCarrierIndices=[52;104;156;208;260]  CyclicPrefixLength=0  Windowing=off  WindowLength=1  OversamplingFactor=1  NumSymbols=1  NumTransmitAntennas=1  SimulateUsing=Interpreted execution
  Rectangular QAM Modulator Baseband : commdigbbndam3/Rectangular QAM Modulator Baseband  M=4096  InType=Bit  Enc=Gray  Mapping=[0:15]  PowType=Min. distance between symbols  MinDist=2  AvgPow=1  PeakPow=1  Ph=0  outDtype=double  outWordLen=16  outUDDataType=sfix(16)  outFracLenMode=Best precision  outFracLen=15  outDataTypeStr=double  outLastDataTypeStr=double
  Out1 : Outport
  wires:
  Rectangular QAM Modulator Baseband/1 -> OFDM Modulator/1
  OFDM Modulator/1 -> Out1/1
  BCH Encoder/1 -> Rectangular QAM Modulator Baseband/1
  In1/1 -> BCH Encoder/1

== system B/4K QAM/MSC13 WiFi Modulation16 ==
  In1 : Inport
  BCH Encoder : commblkcod2/BCH Encoder  n=47040  k=39200  specShortening=off  shortenedK=5  specGenPoly=off  genPoly='X^10 + X^8 + X^5 + X^4 + X^2 + X + 1'  specPrimPoly=off  prPoly='X^4 + X + 1'  specDisableGenCheck=off  specPuncture=off  punctVec=[ones(8,1); zeros(2,1)]
  OFDM Modulator : commofdm/OFDM Modulator  StatePerturbationForJacobian=1.0e-05  FFTLength=4096  NumGuardBandCarriers=[88; 88]  InsertDCNull=off  PilotInputPort=off  PilotCarrierIndices=[52;104;156;208;260]  CyclicPrefixLength=0  Windowing=off  WindowLength=1  OversamplingFactor=1  NumSymbols=1  NumTransmitAntennas=1  SimulateUsing=Interpreted execution
  Rectangular QAM Modulator Baseband : commdigbbndam3/Rectangular QAM Modulator Baseband  M=4096  InType=Bit  Enc=Gray  Mapping=[0:15]  PowType=Min. distance between symbols  MinDist=2  AvgPow=1  PeakPow=1  Ph=0  outDtype=double  outWordLen=16  outUDDataType=sfix(16)  outFracLenMode=Best precision  outFracLen=15  outDataTypeStr=double  outLastDataTypeStr=double
  Out1 : Outport
  wires:
  Rectangular QAM Modulator Baseband/1 -> OFDM Modulator/1
  OFDM Modulator/1 -> Out1/1
  BCH Encoder/1 -> Rectangular QAM Modulator Baseband/1
  In1/1 -> BCH Encoder/1

== system B/4K QAM/MSC13 WiFi Modulation17 ==
  In1 : Inport
  BCH Encoder : commblkcod2/BCH Encoder  n=47040  k=39200  specShortening=off  shortenedK=5  specGenPoly=off  genPoly='X^10 + X^8 + X^5 + X^4 + X^2 + X + 1'  specPrimPoly=off  prPoly='X^4 + X + 1'  specDisableGenCheck=off  specPuncture=off  punctVec=[ones(8,1); zeros(2,1)]
  OFDM Modulator : commofdm/OFDM Modulator  StatePerturbationForJacobian=1.0e-05  FFTLength=4096  NumGuardBandCarriers=[88; 88]  InsertDCNull=off  PilotInputPort=off  PilotCarrierIndices=[52;104;156;208;260]  CyclicPrefixLength=0  Windowing=off  WindowLength=1  OversamplingFactor=1  NumSymbols=1  NumTransmitAntennas=1  SimulateUsing=Interpreted execution
  Rectangular QAM Modulator Baseband : commdigbbndam3/Rectangular QAM Modulator Baseband  M=4096  InType=Bit  Enc=Gray  Mapping=[0:15]  PowType=Min. distance between symbols  MinDist=2  AvgPow=1  PeakPow=1  Ph=0  outDtype=double  outWordLen=16  outUDDataType=sfix(16)  outFracLenMode=Best precision  outFracLen=15  outDataTypeStr=double  outLastDataTypeStr=double
  Out1 : Outport
  wires:
  Rectangular QAM Modulator Baseband/1 -> OFDM Modulator/1
  OFDM Modulator/1 -> Out1/1
  BCH Encoder/1 -> Rectangular QAM Modulator Baseband/1
  In1/1 -> BCH Encoder/1

== system B/4K QAM/MSC13 WiFi Modulation18 ==
  In1 : Inport
  BCH Encoder : commblkcod2/BCH Encoder  n=47040  k=39200  specShortening=off  shortenedK=5  specGenPoly=off  genPoly='X^10 + X^8 + X^5 + X^4 + X^2 + X + 1'  specPrimPoly=off  prPoly='X^4 + X + 1'  specDisableGenCheck=off  specPuncture=off  punctVec=[ones(8,1); zeros(2,1)]
  OFDM Modulator : commofdm/OFDM Modulator  StatePerturbationForJacobian=1.0e-05  FFTLength=4096  NumGuardBandCarriers=[88; 88]  InsertDCNull=off  PilotInputPort=off  PilotCarrierIndices=[52;104;156;208;260]  CyclicPrefixLength=0  Windowing=off  WindowLength=1  OversamplingFactor=1  NumSymbols=1  NumTransmitAntennas=1  SimulateUsing=Interpreted execution
  Rectangular QAM Modulator Baseband : commdigbbndam3/Rectangular QAM Modulator Baseband  M=4096  InType=Bit  Enc=Gray  Mapping=[0:15]  PowType=Min. distance between symbols  MinDist=2  AvgPow=1  PeakPow=1  Ph=0  outDtype=double  outWordLen=16  outUDDataType=sfix(16)  outFracLenMode=Best precision  outFracLen=15  outDataTypeStr=double  outLastDataTypeStr=double
  Out1 : Outport
  wires:
  Rectangular QAM Modulator Baseband/1 -> OFDM Modulator/1
  OFDM Modulator/1 -> Out1/1
  BCH Encoder/1 -> Rectangular QAM Modulator Baseband/1
  In1/1 -> BCH Encoder/1

== system B/4K QAM/MSC13 WiFi Modulation19 ==
  In1 : Inport
  BCH Encoder : commblkcod2/BCH Encoder  n=47040  k=39200  specShortening=off  shortenedK=5  specGenPoly=off  genPoly='X^10 + X^8 + X^5 + X^4 + X^2 + X + 1'  specPrimPoly=off  prPoly='X^4 + X + 1'  specDisableGenCheck=off  specPuncture=off  punctVec=[ones(8,1); zeros(2,1)]
  OFDM Modulator : commofdm/OFDM Modulator  StatePerturbationForJacobian=1.0e-05  FFTLength=4096  NumGuardBandCarriers=[88; 88]  InsertDCNull=off  PilotInputPort=off  PilotCarrierIndices=[52;104;156;208;260]  CyclicPrefixLength=0  Windowing=off  WindowLength=1  OversamplingFactor=1  NumSymbols=1  NumTransmitAntennas=1  SimulateUsing=Interpreted execution
  Rectangular QAM Modulator Baseband : commdigbbndam3/Rectangular QAM Modulator Baseband  M=4096  InType=Bit  Enc=Gray  Mapping=[0:15]  PowType=Min. distance between symbols  MinDist=2  AvgPow=1  PeakPow=1  Ph=0  outDtype=double  outWordLen=16  outUDDataType=sfix(16)  outFracLenMode=Best precision  outFracLen=15  outDataTypeStr=double  outLastDataTypeStr=double
  Out1 : Outport
  wires:
  Rectangular QAM Modulator Baseband/1 -> OFDM Modulator/1
  OFDM Modulator/1 -> Out1/1
  BCH Encoder/1 -> Rectangular QAM Modulator Baseband/1
  In1/1 -> BCH Encoder/1

== system B/4K QAM/MSC13 WiFi Modulation2 ==
  In1 : Inport
  BCH Encoder : commblkcod2/BCH Encoder  n=47040  k=39200  specShortening=off  shortenedK=5  specGenPoly=off  genPoly='X^10 + X^8 + X^5 + X^4 + X^2 + X + 1'  specPrimPoly=off  prPoly='X^4 + X + 1'  specDisableGenCheck=off  specPuncture=off  punctVec=[ones(8,1); zeros(2,1)]
  OFDM Modulator : commofdm/OFDM Modulator  StatePerturbationForJacobian=1.0e-05  FFTLength=4096  NumGuardBandCarriers=[88; 88]  InsertDCNull=off  PilotInputPort=off  PilotCarrierIndices=[52;104;156;208;260]  CyclicPrefixLength=0  Windowing=off  WindowLength=1  OversamplingFactor=1  NumSymbols=1  NumTransmitAntennas=1  SimulateUsing=Interpreted execution
  Rectangular QAM Modulator Baseband : commdigbbndam3/Rectangular QAM Modulator Baseband  M=4096  InType=Bit  Enc=Gray  Mapping=[0:15]  PowType=Min. distance between symbols  MinDist=2  AvgPow=1  PeakPow=1  Ph=0  outDtype=double  outWordLen=16  outUDDataType=sfix(16)  outFracLenMode=Best precision  outFracLen=15  outDataTypeStr=double  outLastDataTypeStr=double
  Out1 : Outport
  wires:
  Rectangular QAM Modulator Baseband/1 -> OFDM Modulator/1
  OFDM Modulator/1 -> Out1/1
  BCH Encoder/1 -> Rectangular QAM Modulator Baseband/1
  In1/1 -> BCH Encoder/1

== system B/4K QAM/MSC13 WiFi Modulation20 ==
  In1 : Inport
  BCH Encoder : commblkcod2/BCH Encoder  n=47040  k=39200  specShortening=off  shortenedK=5  specGenPoly=off  genPoly='X^10 + X^8 + X^5 + X^4 + X^2 + X + 1'  specPrimPoly=off  prPoly='X^4 + X + 1'  specDisableGenCheck=off  specPuncture=off  punctVec=[ones(8,1); zeros(2,1)]
  OFDM Modulator : commofdm/OFDM Modulator  StatePerturbationForJacobian=1.0e-05  FFTLength=4096  NumGuardBandCarriers=[88; 88]  InsertDCNull=off  PilotInputPort=off  PilotCarrierIndices=[52;104;156;208;260]  CyclicPrefixLength=0  Windowing=off  WindowLength=1  OversamplingFactor=1  NumSymbols=1  NumTransmitAntennas=1  SimulateUsing=Interpreted execution
  Rectangular QAM Modulator Baseband : commdigbbndam3/Rectangular QAM Modulator Baseband  M=4096  InType=Bit  Enc=Gray  Mapping=[0:15]  PowType=Min. distance between symbols  MinDist=2  AvgPow=1  PeakPow=1  Ph=0  outDtype=double  outWordLen=16  outUDDataType=sfix(16)  outFracLenMode=Best precision  outFracLen=15  outDataTypeStr=double  outLastDataTypeStr=double
  Out1 : Outport
  wires:
  Rectangular QAM Modulator Baseband/1 -> OFDM Modulator/1
  OFDM Modulator/1 -> Out1/1
  BCH Encoder/1 -> Rectangular QAM Modulator Baseband/1
  In1/1 -> BCH Encoder/1

== system B/4K QAM/MSC13 WiFi Modulation21 ==
  In1 : Inport
  BCH Encoder : commblkcod2/BCH Encoder  n=47040  k=39200  specShortening=off  shortenedK=5  specGenPoly=off  genPoly='X^10 + X^8 + X^5 + X^4 + X^2 + X + 1'  specPrimPoly=off  prPoly='X^4 + X + 1'  specDisableGenCheck=off  specPuncture=off  punctVec=[ones(8,1); zeros(2,1)]
  OFDM Modulator : commofdm/OFDM Modulator  StatePerturbationForJacobian=1.0e-05  FFTLength=4096  NumGuardBandCarriers=[88; 88]  InsertDCNull=off  PilotInputPort=off  PilotCarrierIndices=[52;104;156;208;260]  CyclicPrefixLength=0  Windowing=off  WindowLength=1  OversamplingFactor=1  NumSymbols=1  NumTransmitAntennas=1  SimulateUsing=Interpreted execution
  Rectangular QAM Modulator Baseband : commdigbbndam3/Rectangular QAM Modulator Baseband  M=4096  InType=Bit  Enc=Gray  Mapping=[0:15]  PowType=Min. distance between symbols  MinDist=2  AvgPow=1  PeakPow=1  Ph=0  outDtype=double  outWordLen=16  outUDDataType=sfix(16)  outFracLenMode=Best precision  outFracLen=15  outDataTypeStr=double  outLastDataTypeStr=double
  Out1 : Outport
  wires:
  Rectangular QAM Modulator Baseband/1 -> OFDM Modulator/1
  OFDM Modulator/1 -> Out1/1
  BCH Encoder/1 -> Rectangular QAM Modulator Baseband/1
  In1/1 -> BCH Encoder/1

== system B/4K QAM/MSC13 WiFi Modulation22 ==
  In1 : Inport
  BCH Encoder : commblkcod2/BCH Encoder  n=47040  k=39200  specShortening=off  shortenedK=5  specGenPoly=off  genPoly='X^10 + X^8 + X^5 + X^4 + X^2 + X + 1'  specPrimPoly=off  prPoly='X^4 + X + 1'  specDisableGenCheck=off  specPuncture=off  punctVec=[ones(8,1); zeros(2,1)]
  OFDM Modulator : commofdm/OFDM Modulator  StatePerturbationForJacobian=1.0e-05  FFTLength=4096  NumGuardBandCarriers=[88; 88]  InsertDCNull=off  PilotInputPort=off  PilotCarrierIndices=[52;104;156;208;260]  CyclicPrefixLength=0  Windowing=off  WindowLength=1  OversamplingFactor=1  NumSymbols=1  NumTransmitAntennas=1  SimulateUsing=Interpreted execution
  Rectangular QAM Modulator Baseband : commdigbbndam3/Rectangular QAM Modulator Baseband  M=4096  InType=Bit  Enc=Gray  Mapping=[0:15]  PowType=Min. distance between symbols  MinDist=2  AvgPow=1  PeakPow=1  Ph=0  outDtype=double  outWordLen=16  outUDDataType=sfix(16)  outFracLenMode=Best precision  outFracLen=15  outDataTypeStr=double  outLastDataTypeStr=double
  Out1 : Outport
  wires:
  Rectangular QAM Modulator Baseband/1 -> OFDM Modulator/1
  OFDM Modulator/1 -> Out1/1
  BCH Encoder/1 -> Rectangular QAM Modulator Baseband/1
  In1/1 -> BCH Encoder/1

== system B/4K QAM/MSC13 WiFi Modulation23 ==
  In1 : Inport
  BCH Encoder : commblkcod2/BCH Encoder  n=47040  k=39200  specShortening=off  shortenedK=5  specGenPoly=off  genPoly='X^10 + X^8 + X^5 + X^4 + X^2 + X + 1'  specPrimPoly=off  prPoly='X^4 + X + 1'  specDisableGenCheck=off  specPuncture=off  punctVec=[ones(8,1); zeros(2,1)]
  OFDM Modulator : commofdm/OFDM Modulator  StatePerturbationForJacobian=1.0e-05  FFTLength=4096  NumGuardBandCarriers=[88; 88]  InsertDCNull=off  PilotInputPort=off  PilotCarrierIndices=[52;104;156;208;260]  CyclicPrefixLength=0  Windowing=off  WindowLength=1  OversamplingFactor=1  NumSymbols=1  NumTransmitAntennas=1  SimulateUsing=Interpreted execution
  Rectangular QAM Modulator Baseband : commdigbbndam3/Rectangular QAM Modulator Baseband  M=4096  InType=Bit  Enc=Gray  Mapping=[0:15]  PowType=Min. distance between symbols  MinDist=2  AvgPow=1  PeakPow=1  Ph=0  outDtype=double  outWordLen=16  outUDDataType=sfix(16)  outFracLenMode=Best precision  outFracLen=15  outDataTypeStr=double  outLastDataTypeStr=double
  Out1 : Outport
  wires:
  Rectangular QAM Modulator Baseband/1 -> OFDM Modulator/1
  OFDM Modulator/1 -> Out1/1
  BCH Encoder/1 -> Rectangular QAM Modulator Baseband/1
  In1/1 -> BCH Encoder/1

== system B/4K QAM/MSC13 WiFi Modulation24 ==
  In1 : Inport
  BCH Encoder : commblkcod2/BCH Encoder  n=47040  k=39200  specShortening=off  shortenedK=5  specGenPoly=off  genPoly='X^10 + X^8 + X^5 + X^4 + X^2 + X + 1'  specPrimPoly=off  prPoly='X^4 + X + 1'  specDisableGenCheck=off  specPuncture=off  punctVec=[ones(8,1); zeros(2,1)]
  OFDM Modulator : commofdm/OFDM Modulator  StatePerturbationForJacobian=1.0e-05  FFTLength=4096  NumGuardBandCarriers=[88; 88]  InsertDCNull=off  PilotInputPort=off  PilotCarrierIndices=[52;104;156;208;260]  CyclicPrefixLength=0  Windowing=off  WindowLength=1  OversamplingFactor=1  NumSymbols=1  NumTransmitAntennas=1  SimulateUsing=Interpreted execution
  Rectangular QAM Modulator Baseband : commdigbbndam3/Rectangular QAM Modulator Baseband  M=4096  InType=Bit  Enc=Gray  Mapping=[0:15]  PowType=Min. distance between symbols  MinDist=2  AvgPow=1  PeakPow=1  Ph=0  outDtype=double  outWordLen=16  outUDDataType=sfix(16)  outFracLenMode=Best precision  outFracLen=15  outDataTypeStr=double  outLastDataTypeStr=double
  Out1 : Outport
  wires:
  Rectangular QAM Modulator Baseband/1 -> OFDM Modulator/1
  OFDM Modulator/1 -> Out1/1
  BCH Encoder/1 -> Rectangular QAM Modulator Baseband/1
  In1/1 -> BCH Encoder/1

== system B/4K QAM/MSC13 WiFi Modulation25 ==
  In1 : Inport
  BCH Encoder : commblkcod2/BCH Encoder  n=47040  k=39200  specShortening=off  shortenedK=5  specGenPoly=off  genPoly='X^10 + X^8 + X^5 + X^4 + X^2 + X + 1'  specPrimPoly=off  prPoly='X^4 + X + 1'  specDisableGenCheck=off  specPuncture=off  punctVec=[ones(8,1); zeros(2,1)]
  OFDM Modulator : commofdm/OFDM Modulator  StatePerturbationForJacobian=1.0e-05  FFTLength=4096  NumGuardBandCarriers=[88; 88]  InsertDCNull=off  PilotInputPort=off  PilotCarrierIndices=[52;104;156;208;260]  CyclicPrefixLength=0  Windowing=off  WindowLength=1  OversamplingFactor=1  NumSymbols=1  NumTransmitAntennas=1  SimulateUsing=Interpreted execution
  Rectangular QAM Modulator Baseband : commdigbbndam3/Rectangular QAM Modulator Baseband  M=4096  InType=Bit  Enc=Gray  Mapping=[0:15]  PowType=Min. distance between symbols  MinDist=2  AvgPow=1  PeakPow=1  Ph=0  outDtype=double  outWordLen=16  outUDDataType=sfix(16)  outFracLenMode=Best precision  outFracLen=15  outDataTypeStr=double  outLastDataTypeStr=double
  Out1 : Outport
  wires:
  Rectangular QAM Modulator Baseband/1 -> OFDM Modulator/1
  OFDM Modulator/1 -> Out1/1
  BCH Encoder/1 -> Rectangular QAM Modulator Baseband/1
  In1/1 -> BCH Encoder/1

== system B/4K QAM/MSC13 WiFi Modulation26 ==
  In1 : Inport
  BCH Encoder : commblkcod2/BCH Encoder  n=47040  k=39200  specShortening=off  shortenedK=5  specGenPoly=off  genPoly='X^10 + X^8 + X^5 + X^4 + X^2 + X + 1'  specPrimPoly=off  prPoly='X^4 + X + 1'  specDisableGenCheck=off  specPuncture=off  punctVec=[ones(8,1); zeros(2,1)]
  OFDM Modulator : commofdm/OFDM Modulator  StatePerturbationForJacobian=1.0e-05  FFTLength=4096  NumGuardBandCarriers=[88; 88]  InsertDCNull=off  PilotInputPort=off  PilotCarrierIndices=[52;104;156;208;260]  CyclicPrefixLength=0  Windowing=off  WindowLength=1  OversamplingFactor=1  NumSymbols=1  NumTransmitAntennas=1  SimulateUsing=Interpreted execution
  Rectangular QAM Modulator Baseband : commdigbbndam3/Rectangular QAM Modulator Baseband  M=4096  InType=Bit  Enc=Gray  Mapping=[0:15]  PowType=Min. distance between symbols  MinDist=2  AvgPow=1  PeakPow=1  Ph=0  outDtype=double  outWordLen=16  outUDDataType=sfix(16)  outFracLenMode=Best precision  outFracLen=15  outDataTypeStr=double  outLastDataTypeStr=double
  Out1 : Outport
  wires:
  Rectangular QAM Modulator Baseband/1 -> OFDM Modulator/1
  OFDM Modulator/1 -> Out1/1
  BCH Encoder/1 -> Rectangular QAM Modulator Baseband/1
  In1/1 -> BCH Encoder/1

== system B/4K QAM/MSC13 WiFi Modulation27 ==
  In1 : Inport
  BCH Encoder : commblkcod2/BCH Encoder  n=47040  k=39200  specShortening=off  shortenedK=5  specGenPoly=off  genPoly='X^10 + X^8 + X^5 + X^4 + X^2 + X + 1'  specPrimPoly=off  prPoly='X^4 + X + 1'  specDisableGenCheck=off  specPuncture=off  punctVec=[ones(8,1); zeros(2,1)]
  OFDM Modulator : commofdm/OFDM Modulator  StatePerturbationForJacobian=1.0e-05  FFTLength=4096  NumGuardBandCarriers=[88; 88]  InsertDCNull=off  PilotInputPort=off  PilotCarrierIndices=[52;104;156;208;260]  CyclicPrefixLength=0  Windowing=off  WindowLength=1  OversamplingFactor=1  NumSymbols=1  NumTransmitAntennas=1  SimulateUsing=Interpreted execution
  Rectangular QAM Modulator Baseband : commdigbbndam3/Rectangular QAM Modulator Baseband  M=4096  InType=Bit  Enc=Gray  Mapping=[0:15]  PowType=Min. distance between symbols  MinDist=2  AvgPow=1  PeakPow=1  Ph=0  outDtype=double  outWordLen=16  outUDDataType=sfix(16)  outFracLenMode=Best precision  outFracLen=15  outDataTypeStr=double  outLastDataTypeStr=double
  Out1 : Outport
  wires:
  Rectangular QAM Modulator Baseband/1 -> OFDM Modulator/1
  OFDM Modulator/1 -> Out1/1
  BCH Encoder/1 -> Rectangular QAM Modulator Baseband/1
  In1/1 -> BCH Encoder/1

== system B/4K QAM/MSC13 WiFi Modulation28 ==
  In1 : Inport
  BCH Encoder : commblkcod2/BCH Encoder  n=47040  k=39200  specShortening=off  shortenedK=5  specGenPoly=off  genPoly='X^10 + X^8 + X^5 + X^4 + X^2 + X + 1'  specPrimPoly=off  prPoly='X^4 + X + 1'  specDisableGenCheck=off  specPuncture=off  punctVec=[ones(8,1); zeros(2,1)]
  OFDM Modulator : commofdm/OFDM Modulator  StatePerturbationForJacobian=1.0e-05  FFTLength=4096  NumGuardBandCarriers=[88; 88]  InsertDCNull=off  PilotInputPort=off  PilotCarrierIndices=[52;104;156;208;260]  CyclicPrefixLength=0  Windowing=off  WindowLength=1  OversamplingFactor=1  NumSymbols=1  NumTransmitAntennas=1  SimulateUsing=Interpreted execution
  Rectangular QAM Modulator Baseband : commdigbbndam3/Rectangular QAM Modulator Baseband  M=4096  InType=Bit  Enc=Gray  Mapping=[0:15]  PowType=Min. distance between symbols  MinDist=2  AvgPow=1  PeakPow=1  Ph=0  outDtype=double  outWordLen=16  outUDDataType=sfix(16)  outFracLenMode=Best precision  outFracLen=15  outDataTypeStr=double  outLastDataTypeStr=double
  Out1 : Outport
  wires:
  Rectangular QAM Modulator Baseband/1 -> OFDM Modulator/1
  OFDM Modulator/1 -> Out1/1
  BCH Encoder/1 -> Rectangular QAM Modulator Baseband/1
  In1/1 -> BCH Encoder/1
